simulink model "Induction_Machine"  (R2017a)
settings: Solver=VariableStepAuto  StartTime=0.0  StopTime=10.0  RelTol=1e-3
values from neighbouring files (symbols this model uses):
  Domega = 1    [data1.m]    (also in data2.m; data3.m)
  H = J*(wb)^2/2*(Sb)    (= 4402312961.27)    [data1.m]    (also in data2.m = 292957769866; data3.m = 7.61306125008e+12)
  rpr = 0.228    [data1.m]    (also in data2.m = 0.187; data3.m = 0.022)
  rs = 0.087    [data1.m]    (also in data2.m = 0.262; data3.m = 0.029)
  Tfactor = (3*P)/(2*Sb)    (= 0.000160965794769)    [data1.m]    (also in data2.m = 1.60965794769e-05; data3.m = 3.57701766152e-06)
  V = 460    [data1.m]    (also in data2.m = 2300; data3.m = 2300)
  wb = 2*pi*f    (= 376.991118431)    [data1.m]    (also in data2.m; data3.m)
  xls = 0.302    [data1.m]    (also in data2.m = 1.206; data3.m = 0.226)
  XM = inv(1/xm+1/xls+1/xplr  )    [data1.m]    (also in data2.m; data3.m)
  xplr = 0.302    [data1.m]    (also in data2.m = 1.206; data3.m = 0.226)
  Zb = Vb/Ib    [data1.m]    (also in data2.m; data3.m)
settings Model: Creator=Omid  LastModifiedBy=Omid
settings DataIOCC: ReturnWorkspaceOutputs=on
settings DebuggingCC: UnconnectedInputMsg=none  UnconnectedOutputMsg=none  UnconnectedLineMsg=none
settings SFSimCC: SimUseLocalCustomCode=on
settings RTWCC: RTWUseLocalCustomCode=on

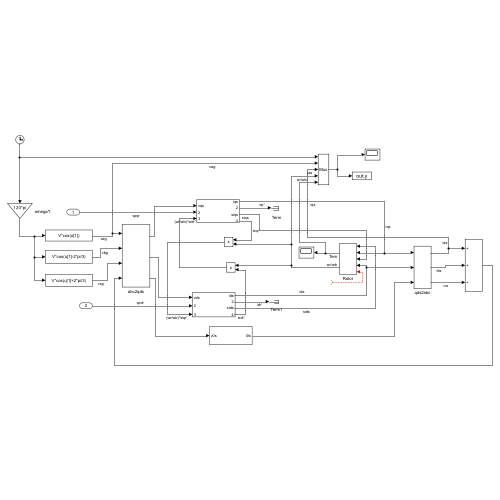
[thumbnail: Simulink's stored preview of the top-level diagram]
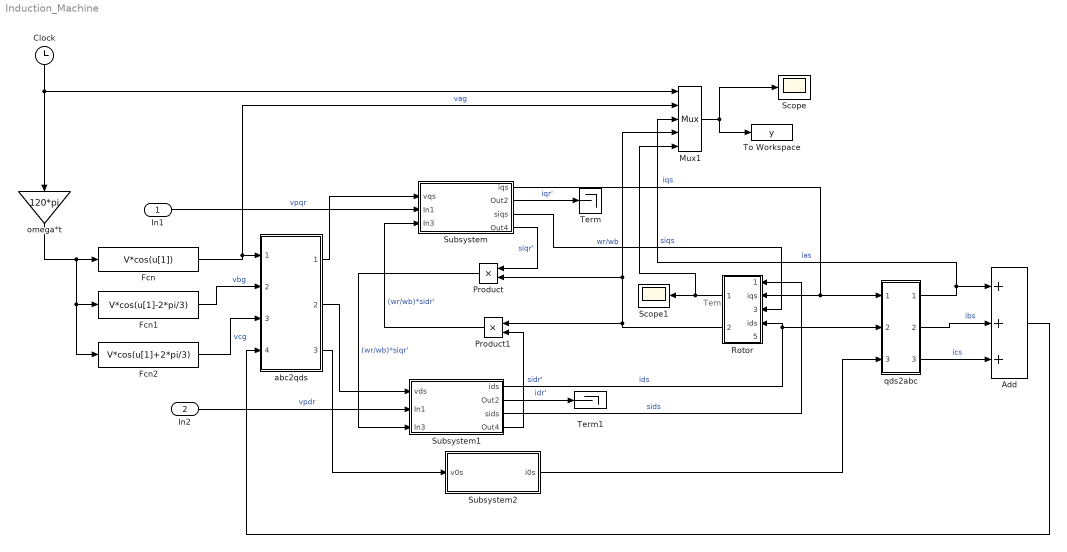
== system Induction_Machine ==
  note: Tem
  In1 : Inport
  In2 : Inport  Port=2
  Add : Sum  Inputs=+++
  Clock : Clock
  Fcn : Fcn  Expr=V*cos(u[1])
  Fcn1 : Fcn  Expr=V*cos(u[1]-2*pi/3)
  Fcn2 : Fcn  Expr=V*cos(u[1]+2*pi/3)
  Mux1 : Mux  Inputs=5
  Product : Product  InputSameDT=on  RndMeth=Zero  SaturateOnIntegerOverflow=on  OutDataTypeStr=Inherit: Same as first input
  Product1 : Product  InputSameDT=on  RndMeth=Zero  SaturateOnIntegerOverflow=on  OutDataTypeStr=Inherit: Same as first input
  Rotor : Subsystem
  Scope : Scope
  Scope1 : Scope
  Subsystem : Subsystem
  Subsystem1 : Subsystem
  Subsystem2 : Subsystem
  Term : Terminator
  Term1 : Terminator
  To Workspace : ToWorkspace  VariableName=y
      settings: MaxDataPoints=80000
  abc2qds : Subsystem
  omega*t : Gain  Gain=120*pi  SaturateOnIntegerOverflow=on  OutDataTypeStr=Inherit: Same as input  ParamDataTypeStr=Inherit: Same as input
  qds2abc : Subsystem
  wires:
  Subsystem1/4(Out4) -> Product1/2  "sidr'"
  Subsystem1/3(sids) -> Rotor/1(sids)  "sids"
  Subsystem/3(siqs) -> Rotor/3(siqs)  "siqs"
  Subsystem/4(Out4) -> Product/1  "siqr'"
  Product1/1 -> Subsystem/3(In3)  "(wr/wb)*sidr'"
  Product/1 -> Subsystem1/3(In3)  "(wr/wb)*siqr'"
  Subsystem/1(iqs) -> Rotor/2(iqs), qds2abc/1(in_iqs)  "iqs"
  Subsystem/2(Out2) -> Term/1  "iqr'"
  Subsystem1/1(ids) -> Rotor/4(ids), qds2abc/2(in_ids)  "ids"
  Subsystem1/2(Out2) -> Term1/1  "idr'"
  Rotor/1(out_Tem) -> Mux1/5, Scope1/1
  Rotor/2(out_wr/wb) -> Product1/1, Product/2, Mux1/4  "wr/wb"
  Subsystem2/1(i0s) -> qds2abc/3(in_i0s)
  abc2qds/1(out_vqs) -> Subsystem/1(vqs)
  abc2qds/2(out_vds) -> Subsystem1/1(vds)
  abc2qds/3(out_v0s) -> Subsystem2/1(v0s)
  qds2abc/1(out_ias) -> Mux1/3, Add/1  "ias"
  qds2abc/2(out_ibs) -> Add/2  "ibs"
  qds2abc/3(out_ics) -> Add/3  "ics"
  Add/1 -> abc2qds/4(ias+ibs+ics)
  Fcn/1 -> Mux1/2, abc2qds/1(in_vag)  "vag"
  Fcn1/1 -> abc2qds/2(in_vbg)  "vbg"
  Fcn2/1 -> abc2qds/3(in_vcg)  "vcg"
  Mux1/1 -> Scope/1, To Workspace/1
  omega*t/1 -> Fcn/1, Fcn1/1, Fcn2/1
  Clock/1 -> omega*t/1, Mux1/1
  In1/1 -> Subsystem/2(In1)  "vpqr"
  In2/1 -> Subsystem1/2(In1)  "vpdr"
  ? -> Rotor/5(Tmech)

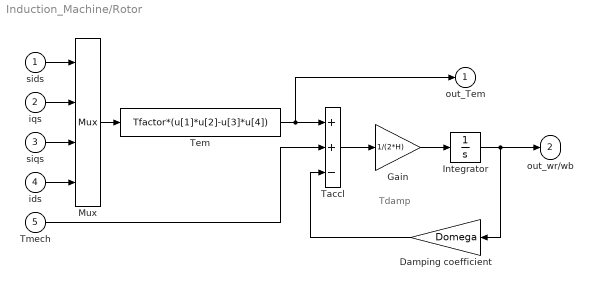
== system Induction_Machine/Rotor ==
  note: Tdamp
  sids : Inport
  iqs : Inport  Port=2
  siqs : Inport  Port=3
  ids : Inport  Port=4
  Tmech : Inport  Port=5
  Damping coefficient : Gain  Gain=Domega  SaturateOnIntegerOverflow=on  OutDataTypeStr=Inherit: Same as input  ParamDataTypeStr=Inherit: Same as input
  Gain : Gain  Gain=1/(2*H)
  Integrator : Integrator
  Mux : Mux
  Taccl : Sum  Inputs=++-  InputSameDT=on  SaturateOnIntegerOverflow=on  OutDataTypeStr=Inherit: Same as first input
  Tem : Fcn  Expr=Tfactor*(u[1]*u[2]-u[3]*u[4])
  out_Tem : Outport  InitialOutput=0
  out_wr/wb : Outport  Port=2  InitialOutput=0
  wires:
  Tmech/1 -> Taccl/2
  Taccl/1 -> Gain/1
  Gain/1 -> Integrator/1
  Tem/1 -> Taccl/1, out_Tem/1
  Integrator/1 -> out_wr/wb/1, Damping coefficient/1
  Damping coefficient/1 -> Taccl/3
  Mux/1 -> Tem/1
  sids/1 -> Mux/1
  iqs/1 -> Mux/2
  siqs/1 -> Mux/3
  ids/1 -> Mux/4

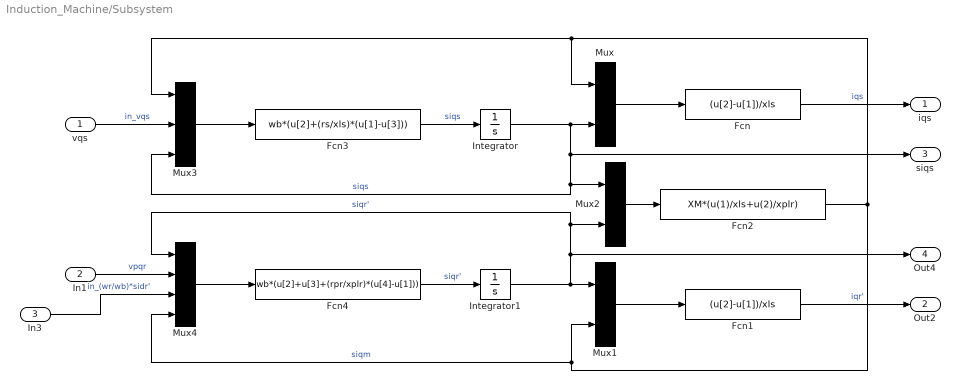
== system Induction_Machine/Subsystem ==
  vqs : Inport
  In1 : Inport  Port=2
  In3 : Inport  Port=3
  Fcn : Fcn  Expr=(u[2]-u[1])/xls
  Fcn1 : Fcn  Expr=(u[2]-u[1])/xls
  Fcn2 : Fcn  Expr=XM*(u(1)/xls+u(2)/xplr)
  Fcn3 : Fcn  Expr=wb*(u[2]+(rs/xls)*(u[1]-u[3]))
  Fcn4 : Fcn  Expr=wb*(u[2]+u[3]+(rpr/xplr)*(u[4]-u[1]))
  Integrator : Integrator
  Integrator1 : Integrator
  Mux : Mux  Inputs=2
  Mux1 : Mux  Inputs=2
  Mux2 : Mux  Inputs=2
  Mux3 : Mux  Inputs=3
  Mux4 : Mux
  iqs : Outport
  Out2 : Outport  Port=2
  siqs : Outport  Port=3
  Out4 : Outport  Port=4
  wires:
  Mux/1 -> Fcn/1
  Integrator/1 -> siqs/1, Mux3/3, Mux2/1, Mux/2  "siqs"
  Mux1/1 -> Fcn1/1
  Integrator1/1 -> Out4/1, Mux4/1, Mux2/2, Mux1/1  "siqr'"
  Mux2/1 -> Fcn2/1
  Fcn2/1 -> Mux/1, Mux3/1, Mux4/4, Mux1/2  "siqm"
  Fcn/1 -> iqs/1  "iqs"
  Fcn1/1 -> Out2/1  "iqr'"
  Mux3/1 -> Fcn3/1
  Mux4/1 -> Fcn4/1
  Fcn4/1 -> Integrator1/1  "siqr'"
  Fcn3/1 -> Integrator/1  "siqs"
  In1/1 -> Mux4/2  "vpqr"
  vqs/1 -> Mux3/2  "in_vqs"
  In3/1 -> Mux4/3  "in_(wr/wb)*sidr'"

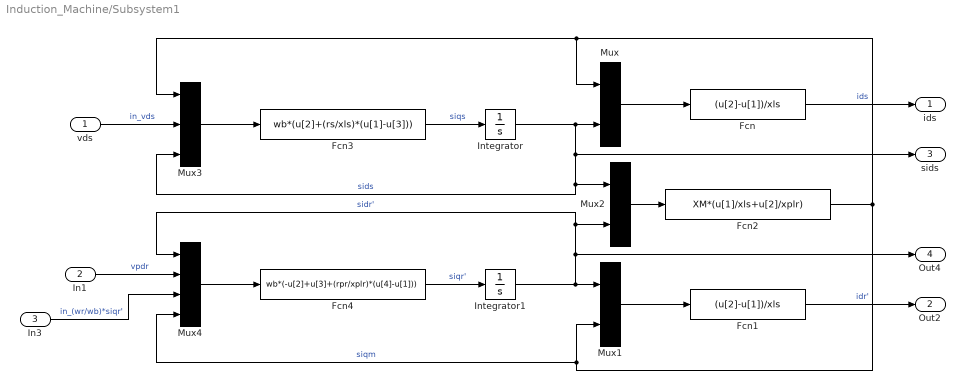
== system Induction_Machine/Subsystem1 ==
  vds : Inport
  In1 : Inport  Port=2
  In3 : Inport  Port=3
  Fcn : Fcn  Expr=(u[2]-u[1])/xls
  Fcn1 : Fcn  Expr=(u[2]-u[1])/xls
  Fcn2 : Fcn  Expr=XM*(u[1]/xls+u[2]/xplr)
  Fcn3 : Fcn  Expr=wb*(u[2]+(rs/xls)*(u[1]-u[3]))
  Fcn4 : Fcn  Expr=wb*(-u[2]+u[3]+(rpr/xplr)*(u[4]-u[1]))
  Integrator : Integrator
  Integrator1 : Integrator
  Mux : Mux  Inputs=2
  Mux1 : Mux  Inputs=2
  Mux2 : Mux  Inputs=2
  Mux3 : Mux  Inputs=3
  Mux4 : Mux
  ids : Outport
  Out2 : Outport  Port=2
  sids : Outport  Port=3
  Out4 : Outport  Port=4
  wires:
  vds/1 -> Mux3/2  "in_vds"
  In1/1 -> Mux4/2  "vpdr"
  Fcn3/1 -> Integrator/1  "siqs"
  Fcn4/1 -> Integrator1/1  "siqr'"
  Mux4/1 -> Fcn4/1
  Mux3/1 -> Fcn3/1
  Fcn1/1 -> Out2/1  "idr'"
  Fcn/1 -> ids/1  "ids"
  Fcn2/1 -> Mux4/4, Mux1/2, Mux3/1, Mux/1  "siqm"
  Mux2/1 -> Fcn2/1
  Integrator1/1 -> Mux1/1, Mux2/2, Mux4/1, Out4/1  "sidr'"
  Mux1/1 -> Fcn1/1
  Integrator/1 -> Mux/2, Mux2/1, Mux3/3, sids/1  "sids"
  Mux/1 -> Fcn/1
  In3/1 -> Mux4/3  "in_(wr/wb)*siqr'"

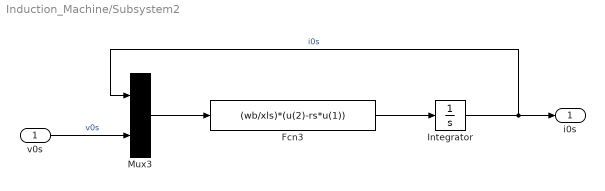
== system Induction_Machine/Subsystem2 ==
  v0s : Inport
  Fcn3 : Fcn  Expr=(wb/xls)*(u(2)-rs*u(1))
  Integrator : Integrator
  Mux3 : Mux  Inputs=2
  i0s : Outport
  wires:
  Integrator/1 -> Mux3/1, i0s/1  "i0s"
  Mux3/1 -> Fcn3/1
  Fcn3/1 -> Integrator/1
  v0s/1 -> Mux3/2  "v0s"

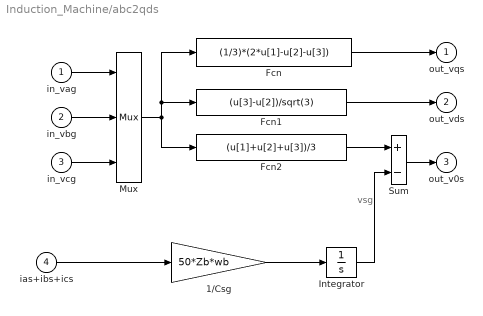
== system Induction_Machine/abc2qds ==
  note: vsg
  in_vag : Inport
  in_vbg : Inport  Port=2
  in_vcg : Inport  Port=3
  ias+ibs+ics : Inport  Port=4
  1/Csg : Gain  Gain=50*Zb*wb  SaturateOnIntegerOverflow=on  OutDataTypeStr=Inherit: Same as input  ParamDataTypeStr=Inherit: Same as input
  Fcn : Fcn  Expr=(1/3)*(2*u[1]-u[2]-u[3])
  Fcn1 : Fcn  Expr=(u[3]-u[2])/sqrt(3)
  Fcn2 : Fcn  Expr=(u[1]+u[2]+u[3])/3
  Integrator : Integrator
  Mux : Mux  Inputs=3
  Sum : Sum  Inputs=+-  InputSameDT=on  SaturateOnIntegerOverflow=on  OutDataTypeStr=Inherit: Same as first input
  out_vqs : Outport  InitialOutput=0
  out_vds : Outport  Port=2  InitialOutput=0
  out_v0s : Outport  Port=3  InitialOutput=0
  wires:
  in_vag/1 -> Mux/1
  in_vbg/1 -> Mux/2
  in_vcg/1 -> Mux/3
  Fcn/1 -> out_vqs/1
  Mux/1 -> Fcn1/1, Fcn/1, Fcn2/1
  Fcn1/1 -> out_vds/1
  Sum/1 -> out_v0s/1
  Fcn2/1 -> Sum/1
  1/Csg/1 -> Integrator/1
  ias+ibs+ics/1 -> 1/Csg/1
  Integrator/1 -> Sum/2

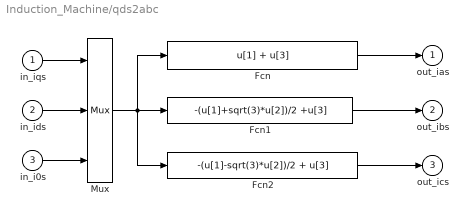
== system Induction_Machine/qds2abc ==
  in_iqs : Inport
  in_ids : Inport  Port=2
  in_i0s : Inport  Port=3
  Fcn : Fcn  Expr=u[1] + u[3]
  Fcn1 : Fcn  Expr=-(u[1]+sqrt(3)*u[2])/2 +u[3]
  Fcn2 : Fcn  Expr=-(u[1]-sqrt(3)*u[2])/2 + u[3]
  Mux : Mux  Inputs=3
  out_ias : Outport  InitialOutput=0
  out_ibs : Outport  Port=2  InitialOutput=0
  out_ics : Outport  Port=3  InitialOutput=0
  wires:
  in_ids/1 -> Mux/2
  in_iqs/1 -> Mux/1
  in_i0s/1 -> Mux/3
  Fcn1/1 -> out_ibs/1
  Fcn/1 -> out_ias/1
  Mux/1 -> Fcn2/1, Fcn1/1, Fcn/1
  Fcn2/1 -> out_ics/1
